simulink model "Q1"  (R2023a)
settings: Solver=VariableStepAuto  StartTime=0.0  StopTime=10  FixedStep=0.01  RelTol=1e-3
settings Model: Creator=DELL  LastModifiedBy=DELL

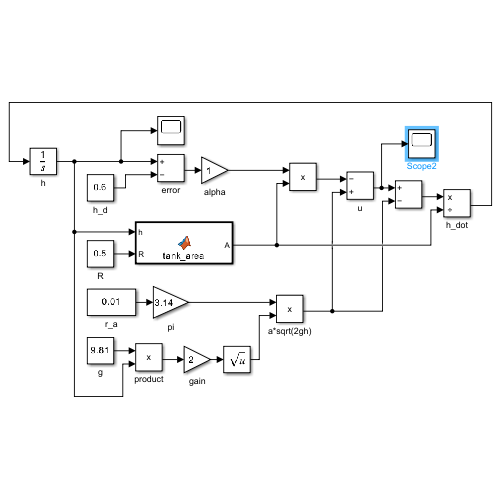
[thumbnail: Simulink's stored preview of the top-level diagram]
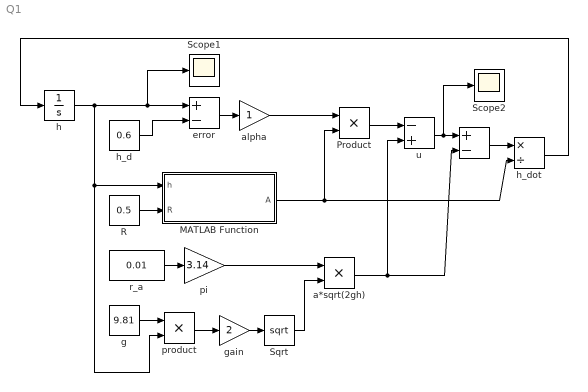
== system Q1 ==
  "  " : Sum  Inputs=+-
  MATLAB Function : MATLAB Function  TreatAsAtomicUnit=on
  Product : Product
  R : Constant  Value=0.5  SampleTime=0.0001
  Scope1 : Scope
  Scope2 : Scope
  Sqrt : Sqrt
  a*sqrt(2gh) : Product
  alpha : Gain
  error : Sum  Inputs=+-
  g : Constant  Value=9.81  SampleTime=0.0001
  gain : Gain  Gain=2
  h : Integrator  InitialCondition=0.1
  h_d : Constant  Value=0.6  SampleTime=0.0001
  h_dot : Product  Inputs=*/
  pi : Gain  Gain=3.14
  product : Product
  r_a : Constant  Value=0.01  SampleTime=0.0001
  u : Sum  Inputs=-+
  wires:
  gain/1 -> Sqrt/1
  r_a/1 -> pi/1
  error/1 -> alpha/1
  product/1 -> gain/1
  pi/1 -> a*sqrt(2gh)/1
  g/1 -> product/1
  R/1 -> MATLAB Function/2(R)
  h_d/1 -> error/2
  Sqrt/1 -> a*sqrt(2gh)/2
  alpha/1 -> Product/1
  MATLAB Function/1(A) -> h_dot/2, Product/2
  Product/1 -> u/1
  a*sqrt(2gh)/1 -> "  "/2, u/2
  u/1 -> Scope2/1, "  "/1
  "  "/1 -> h_dot/1
  h/1 -> product/2, MATLAB Function/1(h), Scope1/1, error/1
  h_dot/1 -> h/1

== matlab function Q1/MATLAB Function ==
  data: h input; A output; R input
function A = tank_area(h, R)
A = pi*h*(2*R-h); % cross-sectional area of spherical tank
end
